simulink model "Simulation"  (R2019b)
settings: Solver=FixedStepAuto  StartTime=0.0  StopTime=5  FixedStep=tau  RelTol=1e-6
values from neighbouring files (symbols this model uses):
  B = 0.3    [main.m]
  b = 0.3    [main.m]
  fullSys = c2d(ss(sys.A,sys.B,sys.C,sys.D,                 'StateName',stateNames,'InputName',inputNames),tau)    [main.m]
  g = 9.81    [main.m]
  K = lqr(sys.A,sys.B_real,Q,R)    [main.m]
  l = 1    [main.m]
  M = 0.75    [main.m]
  m = 0.15    [main.m]
  tau = 0.01    [main.m]
  X0 = [0 deg2rad(0) 0 deg2rad(0)]    [main.m]
undefined symbols (not defined in the file or in its folder): Discrete, Time
libraries: ctrlSharedLib x1, simulink_extras x1
settings Model: Creator=guy-m  LastModifiedBy=Guy

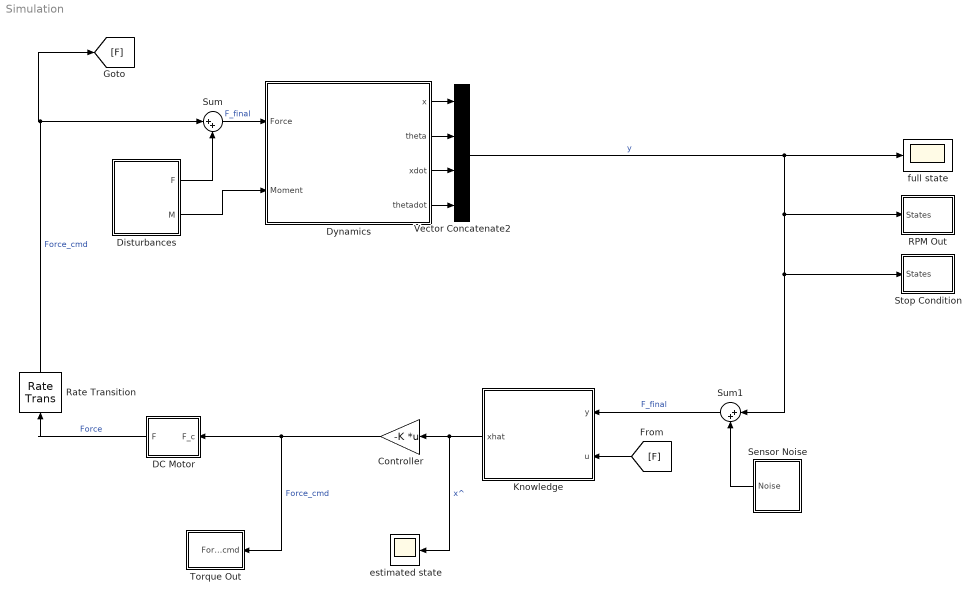
== system Simulation ==
  Controller : Gain  Gain=-K  Multiplication=Matrix(K*u)
  DC Motor : Subsystem
  Disturbances : Subsystem
  Dynamics : Subsystem  Variant=on
  Knowledge : Subsystem  Variant=on
  RPM Out : Subsystem
  Rate Transition : RateTransition  OutPortSampleTime=tau
  Sensor Noise : Subsystem
  Stop Condition : Subsystem
  Sum : Sum  Inputs=|++
  Sum1 : Sum  Inputs=|++
  Torque Out : Subsystem
  Vector Concatenate2 : Concatenate  NumInputs=4
  estimated state : Scope
  full state : Scope
  wires:
  Dynamics/1(x) -> Vector Concatenate2/1
  Dynamics/2(theta) -> Vector Concatenate2/2
  Dynamics/3(xdot) -> Vector Concatenate2/3
  Dynamics/4(thetadot) -> Vector Concatenate2/4
  Vector Concatenate2/1 -> Sum1/1, Stop Condition/1(States), RPM Out/1(States), full state/1  "y"
  Controller/1 -> DC Motor/1(F_c), Torque Out/1(Force_cmd)  "Force_cmd"
  Disturbances/2(M) -> Dynamics/2(Moment)
  Knowledge/1(xhat) -> Controller/1, estimated state/1  "x^"
  DC Motor/1(F) -> Rate Transition/1  "Force"
  [F] -> Knowledge/2(u)
  Sum/1 -> Dynamics/1(Force)  "F_final"
  Disturbances/1(F) -> Sum/2
  Rate Transition/1 -> [F], Sum/1  "Force_cmd"
  Sensor Noise/1(Noise) -> Sum1/2
  Sum1/1 -> Knowledge/1(y)  "F_final"

== system Simulation/DC Motor ==
  F_c : Inport
  Transfer Fcn : TransferFcn  Denominator=[0.01 1]
  F : Outport
  wires:
  F_c/1 -> Transfer Fcn/1
  Transfer Fcn/1 -> F/1

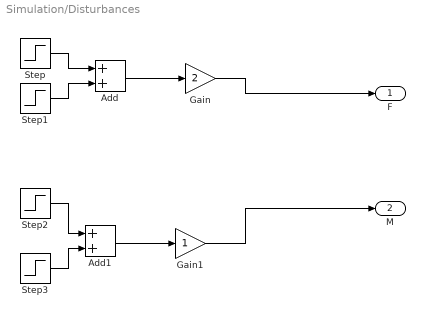
== system Simulation/Disturbances ==
  Add : Sum
  Add1 : Sum
  Gain : Gain  Gain=2
  Gain1 : Gain
  Step : Step  SampleTime=0
  Step1 : Step  Time=1.2  After=-1  SampleTime=0
  Step2 : Step  SampleTime=0
  Step3 : Step  Time=1+0.05  After=-1  SampleTime=0
  F : Outport
  M : Outport  Port=2
  wires:
  Step/1 -> Add/1
  Step1/1 -> Add/2
  Add/1 -> Gain/1
  Step3/1 -> Add1/2
  Step2/1 -> Add1/1
  Add1/1 -> Gain1/1
  Gain/1 -> F/1
  Gain1/1 -> M/1

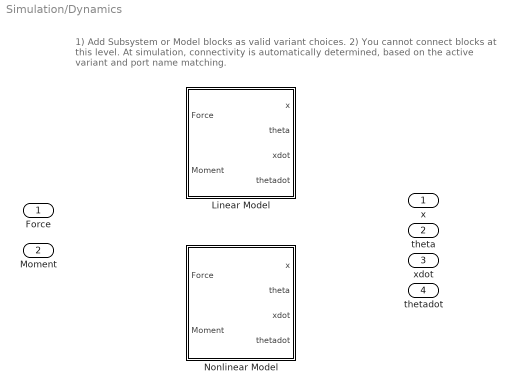
== system Simulation/Dynamics ==
  note: 1) Add Subsystem or Model blocks as valid variant choices.
      | 2) You cannot connect blocks at this level. At simulation, connectivity is automatically
      | determined, based on the active variant and port name matching.
  Force : Inport
  Moment : Inport  Port=2
  Linear Model : Subsystem  VariantControl=linearModel == 1
  Nonlinear Model : Subsystem  VariantControl=linearModel == 0
  x : Outport
  theta : Outport  Port=2
  xdot : Outport  Port=3
  thetadot : Outport  Port=4

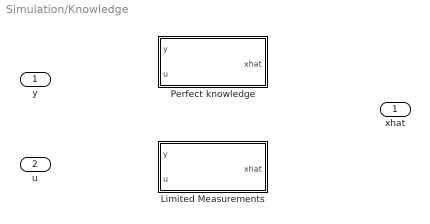
== system Simulation/Knowledge ==
  y : Inport
  u : Inport  Port=2
  Limited Measurements : Subsystem  VariantControl=fullKnowledge == 0
  Perfect knowledge : Subsystem  VariantControl=fullKnowledge == 1
  xhat : Outport

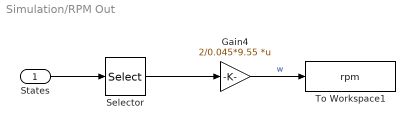
== system Simulation/RPM Out ==
  States : Inport
  Gain4 : Gain  Gain=2/0.045*9.55  Multiplication=Matrix(K*u)
  Selector : Selector  InputPortWidth=4  IndexOptions=Index vector (dialog)  Indices=3  OutputSizes=1
  To Workspace1 : ToWorkspace  VariableName=rpm  SampleTime=-1
  wires:
  Gain4/1 -> To Workspace1/1  "w"
  States/1 -> Selector/1
  Selector/1 -> Gain4/1

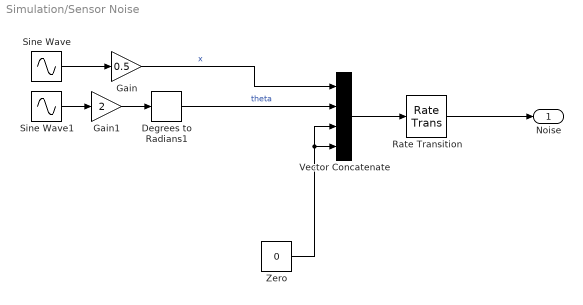
== system Simulation/Sensor Noise ==
  Degrees to Radians1 : simulink_extras/Transformations/Degrees to Radians
  Gain : Gain  Gain=0.5
  Gain1 : Gain  Gain=2
  Rate Transition : RateTransition  OutPortSampleTime=tau
  Sine Wave : Sin  Frequency=100  SampleTime=0
  Sine Wave1 : Sin  Frequency=100  SampleTime=0
  Vector Concatenate : Concatenate  NumInputs=4
  Zero : Constant  Value=0  OutDataTypeStr=Inherit: Inherit via back propagation
  Noise : Outport
  wires:
  Gain1/1 -> Degrees to Radians1/1
  Sine Wave/1 -> Gain/1
  Sine Wave1/1 -> Gain1/1
  Gain/1 -> Vector Concatenate/1  "x"
  Degrees to Radians1/1 -> Vector Concatenate/2  "theta"
  Vector Concatenate/1 -> Rate Transition/1
  Zero/1 -> Vector Concatenate/4, Vector Concatenate/3
  Rate Transition/1 -> Noise/1

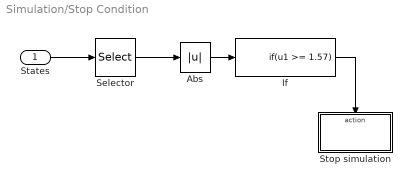
== system Simulation/Stop Condition ==
  States : Inport
  Abs : Abs
  If : If  IfExpression=u1 >= 1.57  ShowElse=off
  Selector : Selector  InputPortWidth=4  IndexOptions=Index vector (dialog)  Indices=2  OutputSizes=1
  Stop simulation : Subsystem  TreatAsAtomicUnit=on
  wires:
  Abs/1 -> If/1
  If/1 -> Stop simulation/Action
  States/1 -> Selector/1
  Selector/1 -> Abs/1

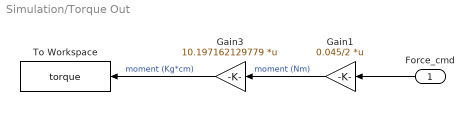
== system Simulation/Torque Out ==
  Force_cmd : Inport
  Gain1 : Gain  Gain=0.045/2  Multiplication=Matrix(K*u)
  Gain3 : Gain  Gain=10.197162129779  Multiplication=Matrix(K*u)
  To Workspace : ToWorkspace  VariableName=torque  SampleTime=-1
  wires:
  Gain3/1 -> To Workspace/1  "moment (Kg*cm)"
  Gain1/1 -> Gain3/1  "moment (Nm)"
  Force_cmd/1 -> Gain1/1

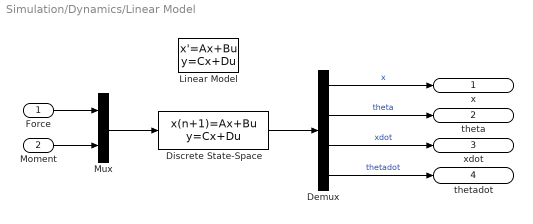
== system Simulation/Dynamics/Linear Model ==
  Force : Inport
  Moment : Inport  Port=2
  Demux : Demux
  Discrete State-Space : DiscreteStateSpace  A=fullSys.A  B=fullSys.B  C=fullSys.C  D=fullSys.D  InitialCondition=X0  SampleTime=tau
  Linear Model : StateSpace  A=fullSys.A  B=fullSys.B  C=fullSys.C  D=fullSys.D  InitialCondition=X0
  Mux : Mux  Inputs=2
  x : Outport
  theta : Outport  Port=2
  xdot : Outport  Port=3
  thetadot : Outport  Port=4
  wires:
  Discrete State-Space/1 -> Demux/1
  Demux/3 -> xdot/1  "xdot"
  Demux/4 -> thetadot/1  "thetadot"
  Demux/1 -> x/1  "x"
  Demux/2 -> theta/1  "theta"
  Mux/1 -> Discrete State-Space/1
  Force/1 -> Mux/1
  Moment/1 -> Mux/2

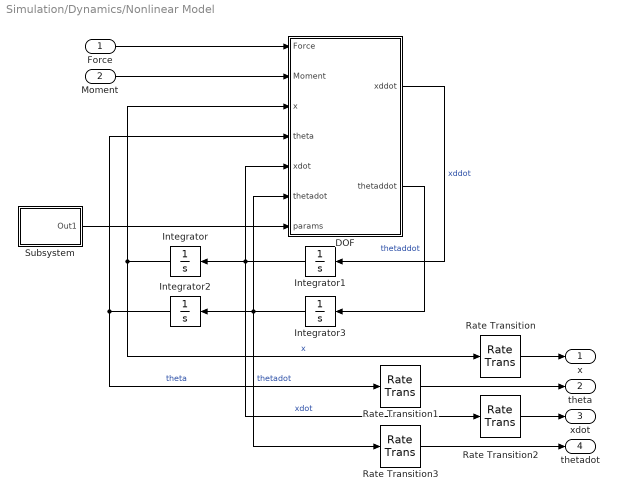
== system Simulation/Dynamics/Nonlinear Model ==
  Force : Inport
  Moment : Inport  Port=2
  DOF : MATLAB Function  TreatAsAtomicUnit=on
  Integrator : Integrator  InitialCondition=X0(1)
  Integrator1 : Integrator  InitialCondition=X0(3)
  Integrator2 : Integrator  InitialCondition=X0(2)
  Integrator3 : Integrator  InitialCondition=X0(4)
  Rate Transition{,1..3} (4 alike) : RateTransition  OutPortSampleTime=tau
  Subsystem : Subsystem
  x : Outport
  theta : Outport  Port=2
  xdot : Outport  Port=3
  thetadot : Outport  Port=4
  wires:
  Force/1 -> DOF/1(Force)
  DOF/1(xddot) -> Integrator1/1  "xddot"
  Integrator/1 -> DOF/3(x), Rate Transition/1  "x"
  Integrator1/1 -> Rate Transition2/1, DOF/5(xdot), Integrator/1  "xdot"
  DOF/2(thetaddot) -> Integrator3/1  "thetaddot"
  Integrator3/1 -> Rate Transition3/1, DOF/6(thetadot), Integrator2/1  "thetadot"
  Integrator2/1 -> DOF/4(theta), Rate Transition1/1  "theta"
  Moment/1 -> DOF/2(Moment)
  Subsystem/1(Out1) -> DOF/7(params)
  Rate Transition/1 -> x/1
  Rate Transition1/1 -> theta/1
  Rate Transition2/1 -> xdot/1
  Rate Transition3/1 -> thetadot/1

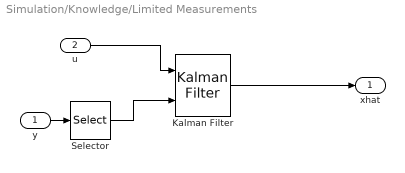
== system Simulation/Knowledge/Limited Measurements ==
  y : Inport
  u : Inport  Port=2
  Kalman Filter : ctrlSharedLib/Kalman Filter  TimeDomain=Discrete-Time  UseCurrentEstimator=on  ModelSource=LTI State-Space Variable  ModelSourceVariable=realSys  A=0.95  B=1  C=1  D=0  NumberOfStates=1  NumberOfInputs=1  NumberOfOutputs=1  InitialEstimateSource=Dialog  X0=0  P0=10  UseK=off  UseGH=off  NumberOfProcessNoiseInputs=1  G=1  TimeInvariantG=on  H=0  TimeInvariantH=on  Q=0.05  TimeInvariantQ=on  R=1  TimeInvariantR=on  N=0  TimeInvariantN=on  AddInputPort=on  AddEnablePort=off  OutputEstimatedY=off  OutputP=off  Ts=-1
      settings: SourceProductBaseCode=CT
  Selector : Selector  InputPortWidth=4  IndexOptions=Index vector (dialog)  Indices=[1 2]  OutputSizes=1
  xhat : Outport
  wires:
  u/1 -> Kalman Filter/1
  y/1 -> Selector/1
  Kalman Filter/1 -> xhat/1
  Selector/1 -> Kalman Filter/2

== system Simulation/Knowledge/Perfect knowledge ==
  y : Inport
  u : Inport  Port=2
  Terminator1 : Terminator
  xhat : Outport
  wires:
  y/1 -> xhat/1
  u/1 -> Terminator1/1

== system Simulation/Stop Condition/Stop simulation ==
  Action Port : ActionPort  ActionPortLabel=if(u1 >= 1.57)
  One : Constant  OutDataTypeStr=Inherit: Inherit via back propagation
  Stop Simulation : Stop
  wires:
  One/1 -> Stop Simulation/1

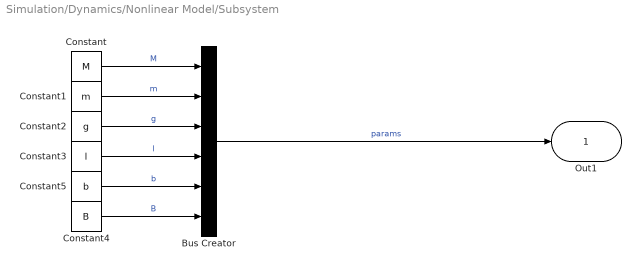
== system Simulation/Dynamics/Nonlinear Model/Subsystem ==
  Bus Creator : BusCreator  Inputs=6  OutDataTypeStr=Bus: params
  Constant : Constant  Value=M
  Constant1 : Constant  Value=m
  Constant2 : Constant  Value=g
  Constant3 : Constant  Value=l
  Constant4 : Constant  Value=B
  Constant5 : Constant  Value=b
  Out1 : Outport  OutDataTypeStr=Bus: params
  wires:
  Constant/1 -> Bus Creator/1  "M"
  Constant1/1 -> Bus Creator/2  "m"
  Constant5/1 -> Bus Creator/5  "b"
  Bus Creator/1 -> Out1/1  "params"
  Constant2/1 -> Bus Creator/3  "g"
  Constant4/1 -> Bus Creator/6  "B"
  Constant3/1 -> Bus Creator/4  "l"

== matlab function Simulation/Dynamics/Nonlinear Model/DOF ==
  data: Force input; Moment input; x input; xddot output size=1; theta input; xdot input; thetadot input; thetaddot output size=1; params input
function [xddot,thetaddot]= fcn(Force,Moment, x,theta,xdot,thetadot, params)


M = params.M;
m = params.m;
l = params.l;
g = params.g;
b = params.b;
B = params.B;

xddot = (- l*m*sin(theta)*thetadot^2 - b*m*cos(theta)*thetadot + Force - B*xdot + Moment*m*cos(theta) + g*m*cos(theta)*sin(theta))/(M + m - m*cos(theta)^2);

thetaddot = (Moment*m + Force*cos(theta) + M*Moment + g*m*sin(theta) - M*b*thetadot - b*m*thetadot - B*xdot*cos(theta) + M*g*sin(theta) - l*m*thetadot^2*cos(theta)*sin(theta))/(l*(M + m - m*cos(theta)^2));
